simulink model "PID"  (R2022a)
settings: Solver=VariableStepAuto  StartTime=0.0  StopTime=1  RelTol=1e-3
settings Model: Creator=FLKU  LastModifiedBy=FLKU

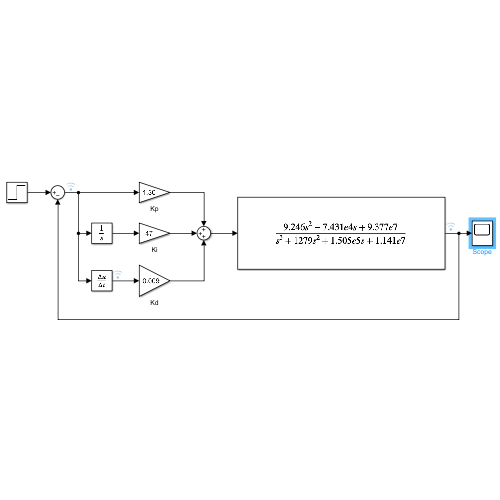
[thumbnail: Simulink's stored preview of the top-level diagram]
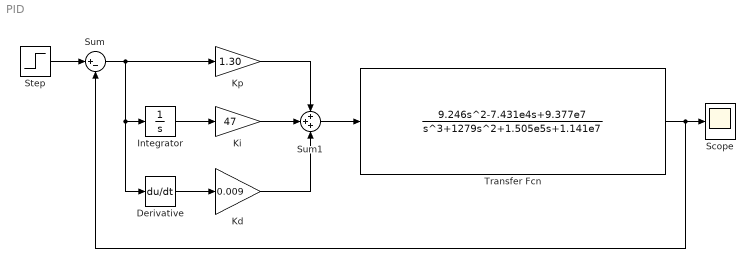
== system PID ==
  Derivative : Derivative
  Integrator : Integrator
  Kd : Gain  Gain=0.009
  Ki : Gain  Gain=47
  Kp : Gain  Gain=1.30
  Scope : Scope
  Step : Step  Time=0  SampleTime=0
  Sum : Sum  Inputs=|+-
  Sum1 : Sum  Inputs=+++
  Transfer Fcn : TransferFcn  Numerator=[9.246 -7.431e4 9.377e7]  Denominator=[1 1279 1.505e5 1.141e7]  ContinuousStateAttributes='position'
  wires:
  Step/1 -> Sum/1
  Sum1/1 -> Transfer Fcn/1
  Kd/1 -> Sum1/3
  Derivative/1 -> Kd/1
  Integrator/1 -> Ki/1
  Kp/1 -> Sum1/1
  Transfer Fcn/1 -> Sum/2, Scope/1
  Sum/1 -> Derivative/1, Integrator/1, Kp/1
  Ki/1 -> Sum1/2
